simulink model "bcd_buoyancy_with_valve_harness"  (R2026a)
settings: Solver=ode23t  StopTime=200  MaxStep=0.1  RelTol=1e-4
libraries: scuba_lib x8, nesl_utility x7, fl_lib x5
settings Model: Creator=grouleau  LastModifiedBy=grouleau

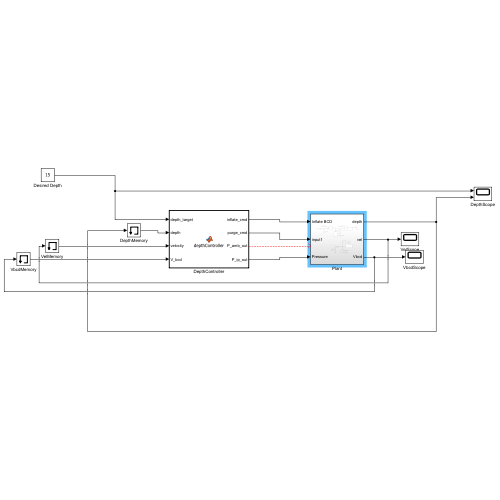
[thumbnail: Simulink's stored preview of the top-level diagram]
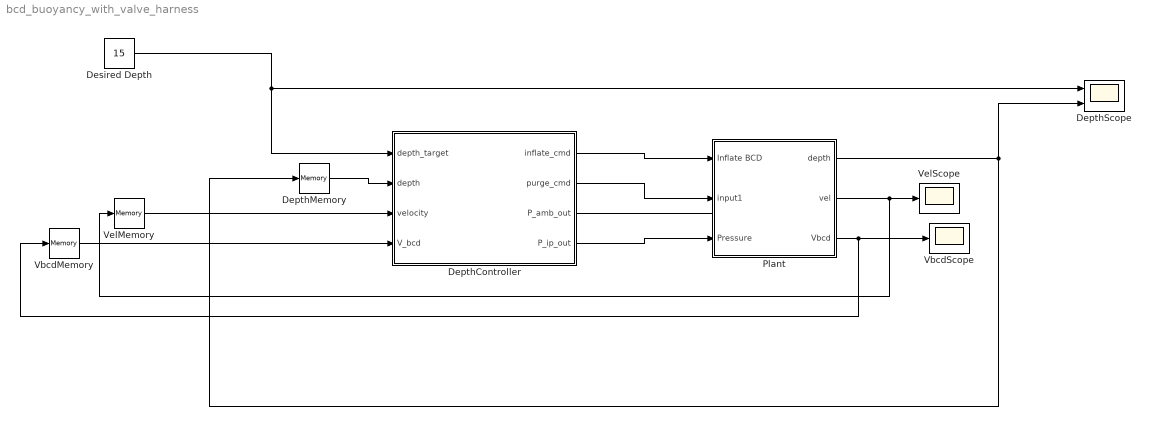
== system bcd_buoyancy_with_valve_harness ==
  DepthController : MATLAB Function  TreatAsAtomicUnit=on
  DepthMemory : Memory  InitialCondition=20
  DepthScope : Scope  NumInputPorts=2
      settings: ActiveDisplayYMinimum=5  ActiveDisplayYMaximum=25
  Desired Depth : Constant  Value=15
  Plant : Subsystem
  VbcdMemory : Memory  InitialCondition=3.9e-4
  VbcdScope : Scope
      settings: ActiveDisplayYMinimum=-0.00011089024738305962  ActiveDisplayYMaximum=0.00099801222644753688
  VelMemory : Memory
  VelScope : Scope
      settings: ActiveDisplayYMinimum=-0.69831849802684554  ActiveDisplayYMaximum=0.59920133742089854
  wires:
  DepthController/3(P_amb_out) -> ?
  VbcdMemory/1 -> DepthController/4(V_bcd)
  VelMemory/1 -> DepthController/3(velocity)
  Plant/3(Vbcd) -> VbcdMemory/1, VbcdScope/1
  Desired Depth/1 -> DepthScope/1, DepthController/1(depth_target)
  DepthMemory/1 -> DepthController/2(depth)
  Plant/1(depth) -> DepthMemory/1, DepthScope/2
  Plant/2(vel) -> VelMemory/1, VelScope/1
  DepthController/1(inflate_cmd) -> Plant/1(Inflate BCD)
  DepthController/2(purge_cmd) -> Plant/2(input1)
  DepthController/4(P_ip_out) -> Plant/3(Pressure)

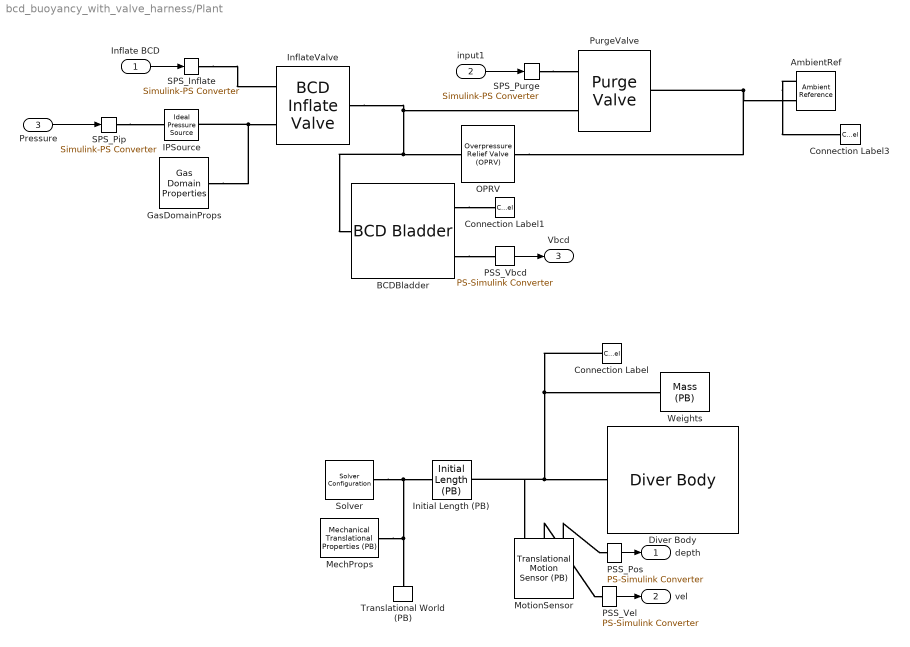
== system bcd_buoyancy_with_valve_harness/Plant ==
  Inflate BCD : Inport
  input1 : Inport  Port=2
  Pressure : Inport  Port=3
  AmbientRef : scuba_lib/gas/elements/Ambient Reference  rho_water=1025 kg/m^3  P_atm=101325 Pa  n_dot_in_specify=off  n_dot_in_priority=None  n_dot_in=0 mol/s  n_dot_in_nominal_specify=off  n_dot_in_nominal_value=1  n_dot_in_nominal_unit=mol/s  f_specify=off  f_priority=None  f=0 N  f_nominal_specify=off  f_nominal_value=1  f_nominal_unit=N
  BCDBladder : scuba_lib/gas/elements/BCD Bladder  V_max=0.015 m^3  n_init=0.048 mol  K_wall=1e7 Pa/m^3  rho_water=1025 kg/m^3  P_atm=101325 Pa  n_dot_in_specify=off  n_dot_in_priority=None  n_dot_in=0 mol/s  n_dot_in_nominal_specify=off  n_dot_in_nominal_value=1  n_dot_in_nominal_unit=mol/s  f_specify=off  f_priority=None  f=0 N  f_nominal_specify=off  f_nominal_value=1  f_nominal_unit=N
  Connection Label : ConnectionLabel  Label=depth
  Connection Label1 : ConnectionLabel  Label=depth
  Connection Label3 : ConnectionLabel  Label=depth
  Diver Body : scuba_lib/Diver Body  V_body=0.065 m^3  rho_body=985 kg/m^3  rho_water=1025 kg/m^3  f_specify=off  f_priority=None  f=0 N  f_nominal_specify=off  f_nominal_value=1  f_nominal_unit=N
  GasDomainProps : scuba_lib/gas/elements/Gas Domain Properties  R_gas=8.314 J/(K*mol)  T=293.15 K  n_dot_thru_specify=off  n_dot_thru_priority=None  n_dot_thru=0 mol/s  n_dot_thru_nominal_specify=off  n_dot_thru_nominal_value=1  n_dot_thru_nominal_unit=mol/s
  IPSource : scuba_lib/gas/elements/Ideal Pressure Source  n_dot_in_specify=off  n_dot_in_priority=None  n_dot_in=0 mol/s  n_dot_in_nominal_specify=off  n_dot_in_nominal_value=1  n_dot_in_nominal_unit=mol/s
  InflateValve : scuba_lib/gas/elements/BCD Inflate Valve  R_open=5e6 Pa*s/mol  n_dot_specify=off  n_dot_priority=None  n_dot=0 mol/s  n_dot_nominal_specify=off  n_dot_nominal_value=1  n_dot_nominal_unit=mol/s
  Initial Length (PB) : fl_lib/Translational/Elements/Initial Length (PB)  length_specify=on  length_priority=High  length=20 m  length_nominal_specify=off  length_nominal_value=1  length_nominal_unit=m  f_specify=off  f_priority=None  f=0 N  f_nominal_specify=off  f_nominal_value=1  f_nominal_unit=N  v_rel_specify=off  v_rel_priority=None  v_rel=0 m/s  v_rel_nominal_specify=off  v_rel_nominal_value=1  v_rel_nominal_unit=m/s
  MechProps : fl_lib/Translational/Utilities/Mechanical Translational Properties (PB)  gravity=9.81 m/s^2  beta=-90 deg
  MotionSensor : fl_lib/Translational/Sensors/Translational Motion Sensor (PB)  reference=foundation.enum.MeasurementReference.absolute  acceleration_port=false  velocity_port=true  position_port=true
  OPRV : scuba_lib/gas/elements/Overpressure Relief Valve (OPRV)  P_crack=20684 Pa  R_open=5000 Pa*s/mol  n_dot_specify=off  n_dot_priority=None  n_dot=0 mol/s  n_dot_nominal_specify=off  n_dot_nominal_value=1  n_dot_nominal_unit=mol/s
  PSS_Pos : nesl_utility/PS-Simulink Converter  PhysicalDomain=network_engine_domain  SubClassName=ps_output  LeftPortType=input  RightPortType=output  PseudoPeriodic=off  Frequencies=[]  VectorFormat=inherit  Unit=inherit  AffineConversion=off
  PSS_Vbcd : nesl_utility/PS-Simulink Converter  PhysicalDomain=network_engine_domain  SubClassName=ps_output  LeftPortType=input  RightPortType=output  PseudoPeriodic=off  Frequencies=[]  VectorFormat=inherit  Unit=inherit  AffineConversion=off
  PSS_Vel : nesl_utility/PS-Simulink Converter  PhysicalDomain=network_engine_domain  SubClassName=ps_output  LeftPortType=input  RightPortType=output  PseudoPeriodic=off  Frequencies=[]  VectorFormat=inherit  Unit=inherit  AffineConversion=off
  PurgeValve : scuba_lib/gas/elements/Purge Valve  R_open=1e4 Pa*s/mol  P_dump=5000 Pa  n_dot_specify=off  n_dot_priority=None  n_dot=0 mol/s  n_dot_nominal_specify=off  n_dot_nominal_value=1  n_dot_nominal_unit=mol/s
  SPS_Inflate : nesl_utility/Simulink-PS Converter  PhysicalDomain=network_engine_domain  SubClassName=ps_input  LeftPortType=input  RightPortType=output  PseudoPeriodic=off  Frequencies=[]  NoiseDistribution=none  NoiseParameters=[]  Unit=1  AffineConversion=off  FilteringAndDerivatives=provide  SimscapeFilterOrder=1  InputFilterTimeConstant=0.001  UdotUserProvided=0
  SPS_Pip : nesl_utility/Simulink-PS Converter  PhysicalDomain=network_engine_domain  SubClassName=ps_input  LeftPortType=input  RightPortType=output  PseudoPeriodic=off  Frequencies=[]  NoiseDistribution=none  NoiseParameters=[]  Unit=1  AffineConversion=off  FilteringAndDerivatives=provide  SimscapeFilterOrder=1  InputFilterTimeConstant=0.001  UdotUserProvided=0
  SPS_Purge : nesl_utility/Simulink-PS Converter  PhysicalDomain=network_engine_domain  SubClassName=ps_input  LeftPortType=input  RightPortType=output  PseudoPeriodic=off  Frequencies=[]  NoiseDistribution=none  NoiseParameters=[]  Unit=1  AffineConversion=off  FilteringAndDerivatives=provide  SimscapeFilterOrder=1  InputFilterTimeConstant=0.001  UdotUserProvided=0
  Solver : nesl_utility/Solver Configuration  PhysicalDomain=network_engine_domain  SubClassName=solver  LeftPortType=input  RightPortType=generic  Tones=[]  Harmonics=[]  SimulateNoise=off  Profile=off  UseLocalSampling=off  EnableSwitchedLinearOptims=on  FrequencyDomain=off  UseCCode=off  RelTol=0.001  AbsTol=0.001  MinStep=1e-09  ToWorkspace=off  RevertToSquareIcSolve=off  NumHomotopyIterations=100  PhasorMode=off  PhasorModeNumHarmonics=1  ConsistencySolver=NEWTON_XTOL_AFTER_FTOL  CanonicalOrdering=CANONICAL  OptimizeIntermediates=OPTIMIZED  IndexReductionMethod=DerivativeReplacement  DoDC=off  ResidualTolerance=1e-09  ConsistencyTolSource=GLOBAL  ConsistencyAbsTol=0.001  ConsistencyRelTol=0.001  ConsistencyTolFactor=0.001  UseLocalSolver=off  LocalSolverChoice=NE_BACKWARD_EULER_ADVANCER  ResolveIndetEquations=on  FunctionEvalNumThread=1  LocalSolverSampleTime=0.001  DoFixedCost=off  MaxNonlinIter=3  MaxModeIter=2  ComputeImpulses=off  ImpulseIterations=2  LinearAlgebra=auto  LinearAlgebraNumThread=0  EquationFormulation=NE_TIME_EF  DelaysMemoryBudget=1024  AutomaticFiltering=on  FilteringTimeConstant=0.001  PartitionStorageMethod=AS_NEEDED  PartitionMemoryBudget=1024  PartitionMethod=ROBUST  MultibodyUseLocalSolver=off  MultibodyLocalSolverChoice=ODE1  MultibodyLocalSolverSampleTime=0.001
  Translational World (PB) : fl_lib/Translational/Elements/Translational World (PB)
  Weights : fl_lib/Translational/Elements/Mass (PB)  mass=3 kg  v_specify=on  v_priority=High  v=0 m/s  v_nominal_specify=off  v_nominal_value=1  v_nominal_unit=m/s  f_acc_specify=off  f_acc_priority=None  f_acc=0 N  f_acc_nominal_specify=off  f_acc_nominal_value=1  f_acc_nominal_unit=N  f_specify=off  f_priority=None  f=0 N  f_nominal_specify=off  f_nominal_value=1  f_nominal_unit=N
  depth : Outport
  vel : Outport  Port=2
  Vbcd : Outport  Port=3
  wires:
  PSS_Pos/1 -> depth/1
  Inflate BCD/1 -> SPS_Inflate/1
  Pressure/1 -> SPS_Pip/1
  PSS_Vel/1 -> vel/1
  input1/1 -> SPS_Purge/1
  PSS_Vbcd/1 -> Vbcd/1
  connections:
  GasDomainProps/LConn1 -- InflateValve/LConn1 -- IPSource/RConn1
  OPRV/RConn1 -- PurgeValve/RConn1 -- AmbientRef/LConn1
  Solver/RConn1 -- Initial Length (PB)/LConn1 -- MechProps/RConn1 -- Translational World (PB)/RConn1
  Connection Label/LConn1 -- Initial Length (PB)/RConn1 -- MotionSensor/RConn1 -- Diver Body/LConn1 -- Weights/LConn1
  InflateValve/RConn1 -- OPRV/LConn1 -- BCDBladder/LConn1 -- PurgeValve/LConn1
  SPS_Pip/RConn1 -- IPSource/LConn1
  BCDBladder/RConn2 -- PSS_Vbcd/LConn1
  SPS_Purge/RConn1 -- PurgeValve/LConn2
  SPS_Inflate/RConn1 -- InflateValve/LConn2
  MotionSensor/RConn3 -- PSS_Pos/LConn1
  MotionSensor/RConn2 -- PSS_Vel/LConn1
  BCDBladder/RConn1 -- Connection Label1/LConn1
  AmbientRef/LConn2 -- Connection Label3/LConn1

== matlab function bcd_buoyancy_with_valve_harness/DepthController ==
  data: depth_target input; inflate_cmd output; depth input; velocity input; V_bcd input; purge_cmd output; P_amb_out output; P_ip_out output
function [inflate_cmd, purge_cmd, P_amb_out, P_ip_out] = depthController(depth_target, depth, velocity, V_bcd)
%% Single-loop proportional valve controller
%% Computes target moles from depth error, outputs proportional valve cmds

P_atm = 101325;
rho_water = 1025;
g = 9.81;
R_gas = 8.314;
T = 293.15;
IP_offset = 10e5;

depth_clamped = max(depth, 0);
P_amb = P_atm + rho_water * g * depth_clamped;
P_ip = P_amb + IP_offset;

P_amb_out = P_amb;
P_ip_out = P_ip;

%% Target BCD moles for neutral buoyancy at target depth
P_target = P_atm + rho_water * g * max(depth_target, 0);
V_neutral = 3.9e-4; %% neutral buoyancy volume at any depth
n_neutral = V_neutral * P_target / (R_gas * T);

%% Depth error -> volume correction
depth_error = depth - depth_target;
Kp = 1e-4; %% m^3 per m depth error
V_correction = Kp * depth_error;
V_target = V_neutral + V_correction;
V_target = max(0, min(0.015, V_target));

%% Convert V_target to moles at current depth
n_target = V_target * P_amb / (R_gas * T);

%% Current moles (from V_bcd at current P_amb)
n_current = V_bcd * P_amb / (R_gas * T);

%% Moles error
n_error = n_current - n_target;

%% Proportional + velocity damping
Kn = 150;   %% gain on moles error -> valve cmd
Kd = 1.5;  %% velocity damping
raw = Kn * n_error - Kd * velocity;

%% Split into inflate/purge with balanced max rates
inflate_max = 0.3;
purge_max = 1.0;

if raw < 0
    inflate_cmd = min(-raw, inflate_max);
    purge_cmd = 0;
else
    inflate_cmd = 0;
    purge_cmd = min(raw, purge_max);
end

end
